simulink model "Algoritmo_Secondo_Ordine"  (R2015a)
settings: Solver=ode45  StartTime=0.0  StopTime=1  RelTol=1e-3
values from neighbouring files (symbols this model uses):
  dif_t = in(9)    [Euler.m]    (also in rob_sic.m = 0.001)
  Kd = kd*eye(4)    [inicia_dinam.m]    (also in rob_sic.m = 50*eye(4))
  Kp = kp*eye(4)    [inicia_dinam.m]    (also in rob_sic.m = 100*eye(4))
settings Model: Creator=TRIANOSAURIO  LastModifiedBy=TRIANOSAURIO

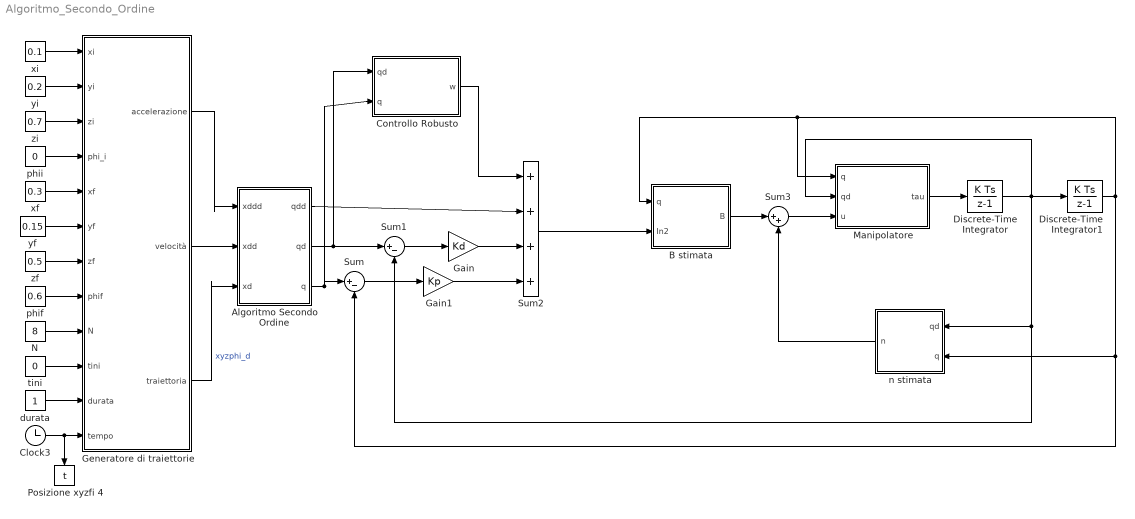
== system Algoritmo_Secondo_Ordine ==
  Algoritmo Secondo Ordine : Subsystem
  B stimata : Subsystem
  Clock3 : Clock
  Controllo Robusto : Subsystem
  Discrete-Time Integrator : DiscreteIntegrator  InitialConditionSetting=State (most efficient)
  Discrete-Time Integrator1 : DiscreteIntegrator  InitialConditionSetting=State (most efficient)
  Gain : Gain  Gain=Kd
  Gain1 : Gain  Gain=Kp
  Generatore di traiettorie : Subsystem
  Manipolatore : Subsystem
  N : Constant  Value=8
  Posizione xyzfi 4 : ToWorkspace  VariableName=t  SampleTime=0.001
  Sum : Sum  Inputs=|+-
  Sum1 : Sum  Inputs=|+-
  Sum2 : Sum  Inputs=++++
  Sum3 : Sum  Inputs=|++
  durata : Constant
  n stimata : Subsystem
  phif : Constant  Value=0.6
  phii : Constant  Value=0
  tini : Constant  Value=0
  xf : Constant  Value=0.3
  xi : Constant  Value=0.1
  yf : Constant  Value=0.15
  yi : Constant  Value=0.2
  zf : Constant  Value=0.5
  zi : Constant  Value=0.7
  wires:
  xi/1 -> Generatore di traiettorie/1(xi)
  yi/1 -> Generatore di traiettorie/2(yi)
  zi/1 -> Generatore di traiettorie/3(zi)
  phii/1 -> Generatore di traiettorie/4(phi_i)
  xf/1 -> Generatore di traiettorie/5(xf)
  yf/1 -> Generatore di traiettorie/6(yf)
  zf/1 -> Generatore di traiettorie/7(zf)
  phif/1 -> Generatore di traiettorie/8(phif)
  N/1 -> Generatore di traiettorie/9(N)
  tini/1 -> Generatore di traiettorie/10(tini)
  durata/1 -> Generatore di traiettorie/11(durata)
  Clock3/1 -> Generatore di traiettorie/12(tempo), Posizione xyzfi 4/1
  Generatore di traiettorie/1(accelerazione) -> Algoritmo Secondo Ordine/1(xddd)
  Generatore di traiettorie/2(velocità) -> Algoritmo Secondo Ordine/2(xdd)
  Generatore di traiettorie/3("traiettoria ") -> Algoritmo Secondo Ordine/3(xd)  "xyzphi_d"
  Algoritmo Secondo Ordine/3(q) -> Controllo Robusto/2(q), Sum/1
  Sum/1 -> Gain1/1
  Algoritmo Secondo Ordine/2(qd) -> Controllo Robusto/1(qd), Sum1/1
  Sum1/1 -> Gain/1
  Gain1/1 -> Sum2/4
  Gain/1 -> Sum2/3
  Algoritmo Secondo Ordine/1(qdd) -> Sum2/2
  Discrete-Time Integrator/1 -> Sum1/2, n stimata/1(qd), Manipolatore/2(qd), Discrete-Time Integrator1/1
  Discrete-Time Integrator1/1 -> Sum/2, n stimata/2(q), Manipolatore/1(q), B stimata/1(q)
  Controllo Robusto/1(w) -> Sum2/1
  n stimata/1(n) -> Sum3/2
  Sum3/1 -> Manipolatore/3(u)
  Manipolatore/1(tau) -> Discrete-Time Integrator/1
  Sum2/1 -> B stimata/2(In2)
  B stimata/1(B) -> Sum3/1

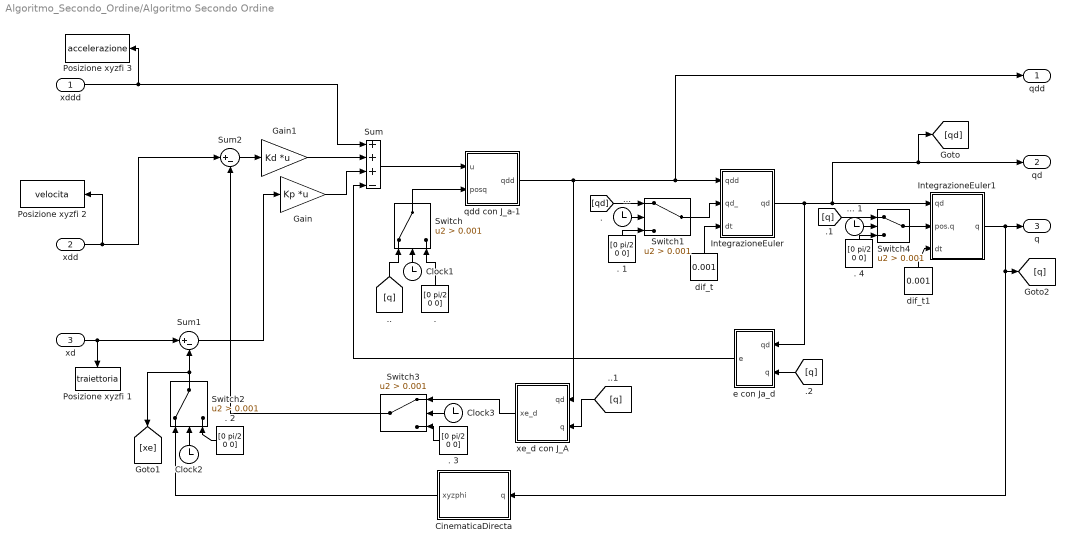
== system Algoritmo_Secondo_Ordine/Algoritmo Secondo Ordine ==
  xddd : Inport
  xdd : Inport  Port=2
  xd : Inport  Port=3
  . {,1..4} (5 alike) : Constant  Value=[0 pi/2 0 0]
  "... " : Clock
  ... 1 : Clock
  CinematicaDirecta : Subsystem
  Clock1 : Clock
  Clock2 : Clock
  Clock3 : Clock
  Gain : Gain  Gain=Kp  Multiplication=Matrix(K*u)
  Gain1 : Gain  Gain=Kd  Multiplication=Matrix(K*u)
  IntegrazioneEuler : Subsystem
  IntegrazioneEuler1 : Subsystem
  Posizione xyzfi 1 : ToWorkspace  VariableName=traiettoria  SampleTime=dif_t
  Posizione xyzfi 2 : ToWorkspace  VariableName=velocita  SampleTime=dif_t
  Posizione xyzfi 3 : ToWorkspace  VariableName=accelerazione  SampleTime=dif_t
  Sum : Sum  Inputs=+++-
  Sum1 : Sum  Inputs=|+-
  Sum2 : Sum  Inputs=|+-
  Switch{,1..4} (5 alike) : Switch  Criteria=u2 > Threshold  Threshold=0.001
  dif_t : Constant  Value=0.001
  dif_t1 : Constant  Value=0.001
  e con Ja_d : Subsystem
  qdd con J_a-1 : Subsystem
  xe_d con J_A : Subsystem
  qdd : Outport
  qd : Outport  Port=2
  q : Outport  Port=3
  wires:
  [qd] -> Switch1/1
  Switch2/1 -> [xe], Sum1/2
  CinematicaDirecta/1(xyzphi) -> Switch2/1
  Clock1/1 -> Switch/2
  Clock2/1 -> Switch2/2
  . 2/1 -> Switch2/3
  . 1/1 -> Switch1/3
  dif_t/1 -> IntegrazioneEuler/3(dt)
  [q] -> Switch/1
  "... "/1 -> Switch1/2
  Sum1/1 -> Gain/1
  Sum/1 -> qdd con J_a-1/1(u)
  qdd con J_a-1/1(qdd) -> xe_d con J_A/1(qd), IntegrazioneEuler/1(qdd), qdd/1
  Switch/1 -> qdd con J_a-1/2(posq)
  Switch1/1 -> IntegrazioneEuler/2(qd_)
  ". "/1 -> Switch/3
  xd/1 -> Sum1/1, Posizione xyzfi 1/1
  xdd/1 -> Posizione xyzfi 2/1, Sum2/1
  [q] -> xe_d con J_A/2(q)
  Gain/1 -> Sum/3
  Sum2/1 -> Gain1/1
  Gain1/1 -> Sum/2
  xddd/1 -> Posizione xyzfi 3/1, Sum/1
  Clock3/1 -> Switch3/2
  . 3/1 -> Switch3/3
  xe_d con J_A/1(xe_d) -> Switch3/1
  Switch3/1 -> Sum2/2
  IntegrazioneEuler/1(qd) -> e con Ja_d/1(qd), [qd], qd/1, IntegrazioneEuler1/1(qd)
  [q] -> Switch4/1
  . 4/1 -> Switch4/3
  ... 1/1 -> Switch4/2
  Switch4/1 -> IntegrazioneEuler1/2(pos.q)
  dif_t1/1 -> IntegrazioneEuler1/3(dt)
  IntegrazioneEuler1/1(q) -> CinematicaDirecta/1(q), [q], q/1
  [q] -> e con Ja_d/2(q)
  e con Ja_d/1(e) -> Sum/4

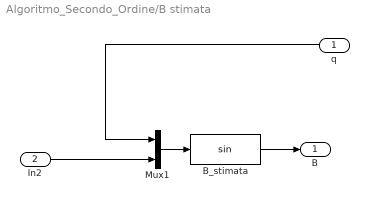
== system Algoritmo_Secondo_Ordine/B stimata ==
  q : Inport
  In2 : Inport  Port=2
  "B_stimata " : MATLABFcn
  Mux1 : Mux  Inputs=2
  B : Outport
  wires:
  "B_stimata "/1 -> B/1
  Mux1/1 -> "B_stimata "/1
  In2/1 -> Mux1/2
  q/1 -> Mux1/1

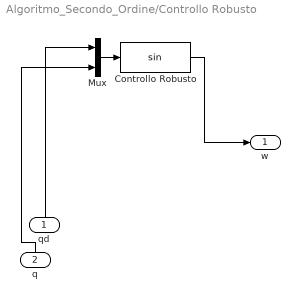
== system Algoritmo_Secondo_Ordine/Controllo Robusto ==
  qd : Inport
  q : Inport  Port=2
  Controllo Robusto : MATLABFcn
  Mux : Mux  Inputs=2
  w : Outport
  wires:
  Mux/1 -> Controllo Robusto/1
  Controllo Robusto/1 -> w/1
  q/1 -> Mux/2
  qd/1 -> Mux/1

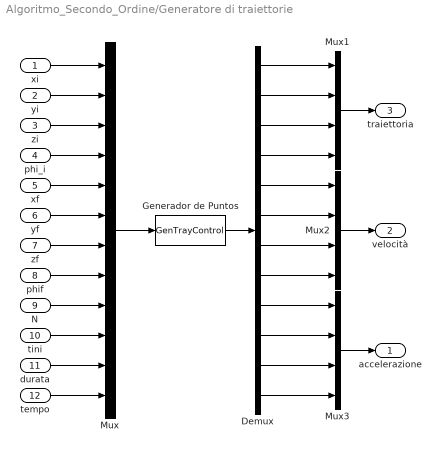
== system Algoritmo_Secondo_Ordine/Generatore di traiettorie ==
  xi : Inport
  yi : Inport  Port=2
  zi : Inport  Port=3
  phi_i : Inport  Port=4
  xf : Inport  Port=5
  yf : Inport  Port=6
  zf : Inport  Port=7
  phif : Inport  Port=8
  N : Inport  Port=9
  tini : Inport  Port=10
  durata : Inport  Port=11
  tempo : Inport  Port=12
  Demux : Demux  Outputs=12
  Generador de Puntos : MATLABFcn  MATLABFcn=GenTrayControl  OutputDimensions=12
  Mux : Mux  Inputs=12
  Mux1 : Mux
  Mux2 : Mux
  Mux3 : Mux
  accelerazione : Outport
  velocità : Outport  Port=2
  "traiettoria " : Outport  Port=3
  wires:
  Mux/1 -> Generador de Puntos/1
  xi/1 -> Mux/1
  yi/1 -> Mux/2
  zi/1 -> Mux/3
  phi_i/1 -> Mux/4
  xf/1 -> Mux/5
  yf/1 -> Mux/6
  zf/1 -> Mux/7
  phif/1 -> Mux/8
  N/1 -> Mux/9
  tini/1 -> Mux/10
  durata/1 -> Mux/11
  tempo/1 -> Mux/12
  Generador de Puntos/1 -> Demux/1
  Mux1/1 -> "traiettoria "/1
  Mux2/1 -> velocità/1
  Mux3/1 -> accelerazione/1
  Demux/12 -> Mux3/4
  Demux/11 -> Mux3/3
  Demux/10 -> Mux3/2
  Demux/9 -> Mux3/1
  Demux/8 -> Mux2/4
  Demux/7 -> Mux2/3
  Demux/6 -> Mux2/2
  Demux/5 -> Mux2/1
  Demux/4 -> Mux1/4
  Demux/1 -> Mux1/1
  Demux/2 -> Mux1/2
  Demux/3 -> Mux1/3

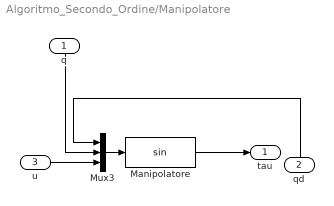
== system Algoritmo_Secondo_Ordine/Manipolatore ==
  q : Inport
  qd : Inport  Port=2
  u : Inport  Port=3
  Manipolatore : MATLABFcn
  Mux3 : Mux  Inputs=3
  tau : Outport
  wires:
  u/1 -> Mux3/3
  Mux3/1 -> Manipolatore/1
  q/1 -> Mux3/2
  qd/1 -> Mux3/1
  Manipolatore/1 -> tau/1

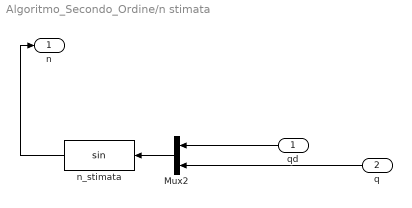
== system Algoritmo_Secondo_Ordine/n stimata ==
  qd : Inport
  q : Inport  Port=2
  Mux2 : Mux  Inputs=2
  "n_stimata " : MATLABFcn
  n : Outport
  wires:
  q/1 -> Mux2/2
  qd/1 -> Mux2/1
  "n_stimata "/1 -> n/1
  Mux2/1 -> "n_stimata "/1

== system Algoritmo_Secondo_Ordine/Algoritmo Secondo Ordine/CinematicaDirecta ==
  q : Inport
  Interpreted MATLAB Function : MATLABFcn  MATLABFcn=CinematicaDirecta
  xyzphi : Outport
  wires:
  q/1 -> Interpreted MATLAB Function/1
  Interpreted MATLAB Function/1 -> xyzphi/1

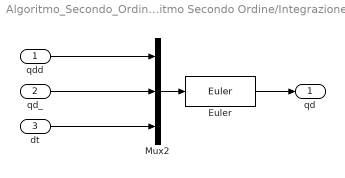
== system Algoritmo_Secondo_Ordine/Algoritmo Secondo Ordine/IntegrazioneEuler ==
  qdd : Inport
  qd_ : Inport  Port=2
  dt : Inport  Port=3
  Euler : MATLABFcn  MATLABFcn=Euler
  Mux2 : Mux  Inputs=3
  qd : Outport
  wires:
  Euler/1 -> qd/1
  qdd/1 -> Mux2/1
  Mux2/1 -> Euler/1
  qd_/1 -> Mux2/2
  dt/1 -> Mux2/3

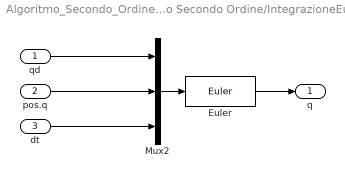
== system Algoritmo_Secondo_Ordine/Algoritmo Secondo Ordine/IntegrazioneEuler1 ==
  qd : Inport
  pos.q : Inport  Port=2
  dt : Inport  Port=3
  Euler : MATLABFcn  MATLABFcn=Euler
  Mux2 : Mux  Inputs=3
  q : Outport
  wires:
  dt/1 -> Mux2/3
  pos.q/1 -> Mux2/2
  Mux2/1 -> Euler/1
  qd/1 -> Mux2/1
  Euler/1 -> q/1

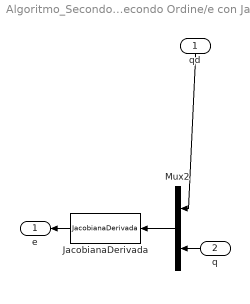
== system Algoritmo_Secondo_Ordine/Algoritmo Secondo Ordine/e con Ja_d ==
  qd : Inport
  q : Inport  Port=2
  JacobianaDerivada : MATLABFcn  MATLABFcn=JacobianaDerivada
  Mux2 : Mux  Inputs=2
  e : Outport
  wires:
  q/1 -> Mux2/2
  JacobianaDerivada/1 -> e/1
  qd/1 -> Mux2/1
  Mux2/1 -> JacobianaDerivada/1

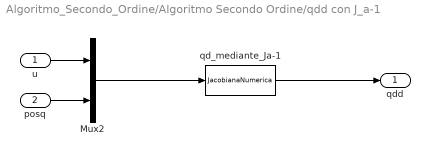
== system Algoritmo_Secondo_Ordine/Algoritmo Secondo Ordine/qdd con J_a-1 ==
  u : Inport
  posq : Inport  Port=2
  Mux2 : Mux  Inputs=2
  qd_mediante_Ja-1 : MATLABFcn  MATLABFcn=JacobianaNumerica
  qdd : Outport
  wires:
  qd_mediante_Ja-1/1 -> qdd/1
  Mux2/1 -> qd_mediante_Ja-1/1
  u/1 -> Mux2/1
  posq/1 -> Mux2/2

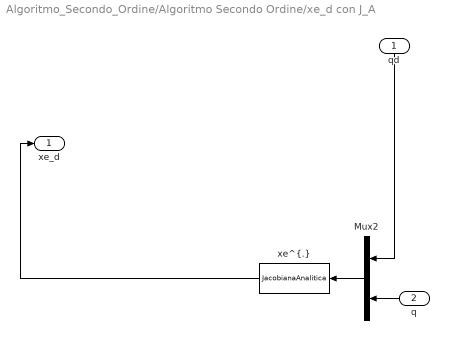
== system Algoritmo_Secondo_Ordine/Algoritmo Secondo Ordine/xe_d con J_A ==
  qd : Inport
  q : Inport  Port=2
  Mux2 : Mux  Inputs=2
  "xe^{.}" : MATLABFcn  MATLABFcn=JacobianaAnalitica
  xe_d : Outport
  wires:
  q/1 -> Mux2/2
  Mux2/1 -> "xe^{.}"/1
  qd/1 -> Mux2/1
  "xe^{.}"/1 -> xe_d/1
